simulink model "Q6"  (R2020b)
settings: Solver=VariableStepAuto  StartTime=0.0  StopTime=10.0  RelTol=1e-3
settings Model: Creator=HP  LastModifiedBy=HP

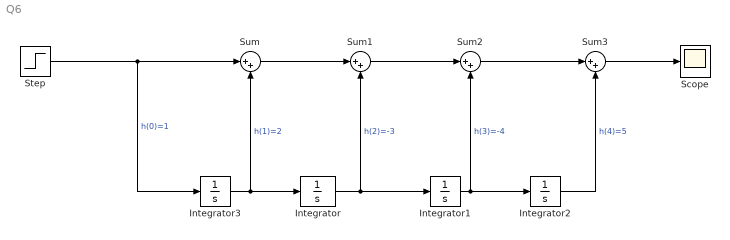
== system Q6 ==
  Integrator{,1..3} (4 alike) : Integrator
  Scope : Scope
  Step : Step  SampleTime=0
  Sum{,1..3} (4 alike) : Sum  Inputs=|++
  wires:
  Integrator2/1 -> Sum3/2  "h(4)=5"
  Step/1 -> Integrator3/1, Sum/1  "h(0)=1"
  Sum1/1 -> Sum2/1
  Integrator3/1 -> Sum/2, Integrator/1  "h(1)=2"
  Integrator1/1 -> Integrator2/1, Sum2/2  "h(3)=-4"
  Sum3/1 -> Scope/1
  Sum/1 -> Sum1/1
  Sum2/1 -> Sum3/1
  Integrator/1 -> Sum1/2, Integrator1/1  "h(2)=-3"
